simulink model "fig9_53and54"  (Simulink 4.00)
settings: Solver=ode23  SolverMode=SingleTasking  StartTime=0.0  StopTime=20.0  RelTol=1e-3  AbsTol=1e-5
settings Model: LastModifiedBy=abbas  LimitDataPoints=off  ExtModeTrigMode=oneshot  ExtModeArmWhenConnect=off  BlockReductionOpt=off

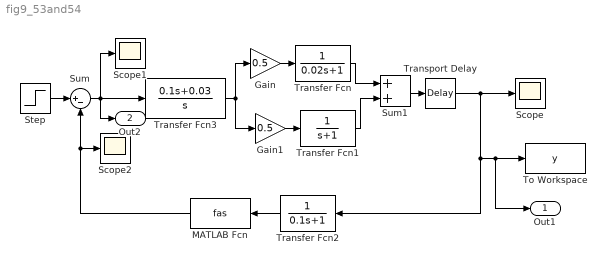
== system fig9_53and54 ==
  Gain : Gain  Gain=0.5  Multiplication=Element-wise(K.*u)  SaturateOnIntegerOverflow=on
  Gain1 : Gain  Gain=0.5  Multiplication=Element-wise(K.*u)  SaturateOnIntegerOverflow=on
  MATLAB Fcn : MATLABFcn  Orientation=left  MATLABFcn=fas  OutputDimensions=1  OutputSignalType=auto  Output1D=on
  Scope : Scope
      settings: TickLabels=on  TimeRange=auto  YMin=-5  YMax=5  SaveToWorkspace=off  SaveName=ScopeData  DataFormat=Array  LimitDataPoints=on  MaxDataPoints=5000
  Scope1 : Scope
      settings: TickLabels=on  TimeRange=auto  YMin=-5  YMax=5  SaveToWorkspace=off  SaveName=ScopeData  DataFormat=Array  LimitDataPoints=on  MaxDataPoints=5000
  Scope2 : Scope
      settings: TickLabels=on  TimeRange=auto  YMin=-5  YMax=5  SaveToWorkspace=off  SaveName=ScopeData  DataFormat=Array  LimitDataPoints=on  MaxDataPoints=5000
  Step : Step  Time=0  Before=0  After=0.5  SampleTime=-1
  Sum : Sum  Inputs=|+-  SaturateOnIntegerOverflow=on
  Sum1 : Sum  Inputs=++  SaturateOnIntegerOverflow=on
  To Workspace : ToWorkspace  VariableName=y  SampleTime=-1  SaveFormat=Array
  Transfer Fcn : TransferFcn  Numerator=[1]  Denominator=[0.02 1]  Realization=auto  AbsoluteTolerance=auto
  Transfer Fcn1 : TransferFcn  Numerator=[1]  Denominator=[1 1]  Realization=auto  AbsoluteTolerance=auto
  Transfer Fcn2 : TransferFcn  Orientation=left  Numerator=[1]  Denominator=[0.1 1]  Realization=auto  AbsoluteTolerance=auto
  Transfer Fcn3 : TransferFcn  Numerator=[0.1 0.03]  Denominator=[1 0]  Realization=auto  AbsoluteTolerance=auto
  Transport Delay : TransportDelay  DelayTime=0.2  InitialInput=0  BufferSize=1024  PadeOrder=0
  Out1 : Outport  Port=1
  Out2 : Outport  Port=2
  wires:
  Transfer Fcn1/1 -> Sum1/2
  Sum1/1 -> Transport Delay/1
  Transport Delay/1 -> Scope/1, Transfer Fcn2/1, To Workspace/1, Out1/1
  Transfer Fcn/1 -> Sum1/1
  Gain/1 -> Transfer Fcn/1
  Transfer Fcn3/1 -> Gain/1, Gain1/1
  Gain1/1 -> Transfer Fcn1/1
  Transfer Fcn2/1 -> MATLAB Fcn/1
  MATLAB Fcn/1 -> Scope2/1, Sum/2
  Step/1 -> Sum/1
  Sum/1 -> Transfer Fcn3/1, Scope1/1, Out2/1
